simulink model "Project_sim"  (R2025b)
settings: Solver=ode4  StartTime=0.0  StopTime=2*T  FixedStep=0.1  RelTol=1e-3
values from neighbouring files (symbols this model uses):
  a = 3000+R_E    [RUN_ME.m]
  A_0 = [cos(th0+epsilon1) sin(th0+epsilon1) 0; -sin(th0+epsilon1) cos(th0+epsilon1) 0; 0 0 1]*    [1 0 0; 0 cos(i+epsilon2) sin(i+epsilon2); 0 -sin(i+epsilon2) cos(i+epsilon2)]    [RUN_ME.m]
  alpha1 = 0.72    [RUN_ME.m]
  alpha_G0 = 0    [RUN_ME.m]
  AU = astroConstants(2)    [RUN_ME.m]
  b_gyro = deg2rad(0.01*rand(1))    [RUN_ME.m]
  b_mag = 15e-9    (= 1.5e-08)    [RUN_ME.m]
  b_sun = deg2rad(0.1*rand(1))    [RUN_ME.m]
  c_time = 100    [RUN_ME.m]
  D = zeros(3)    [RUN_ME.m]
  den_cz_mag = double(sym2poly(den8_z_mag))    [RUN_ME.m]
  den_cz_sun = double(sym2poly(den8_z_sun))    [RUN_ME.m]
  e = 0.2    [RUN_ME.m]
  epsilon = astroConstants(8)    [RUN_ME.m]
  g_IGRF = [ ... (first row only)    [RUN_ME.m]
  gyro_delay = 1    [RUN_ME.m]
  gyro_mounting = eye(3)    [RUN_ME.m]
  h_IGRF = [ ... (first row only)    [RUN_ME.m]
  I = [Ix 0 0; 0 Iy 0; 0 0 Iz]    [RUN_ME.m]
  i = deg2rad(30)    [RUN_ME.m]
  j_B = [0.01; 0.05; 0.01]    [RUN_ME.m]
  K = place(A, -B, a_controlled)    [RUN_ME.m]
  k1 = 20e-4    (= 0.002)    [RUN_ME.m]
  k1_tilde = 5e-4    (= 0.0005)    [RUN_ME.m]
  k2 = 2e-4    (= 0.0002)    [RUN_ME.m]
  Mis_gyro = deg2rad(0.1*rand(3,1))    [RUN_ME.m]
  Mis_mag = deg2rad(0.1*rand(3,1))    [RUN_ME.m]
  Mis_sun = deg2rad(0.1*rand(3,1))    [RUN_ME.m]
  mu = astroConstants(13)    [RUN_ME.m]
  n = sqrt(mu/a^3)    [RUN_ME.m]
  noise_density_mag = 16e-9    (= 1.6e-08)    [RUN_ME.m]
  Nonorthog_err_gyro = deg2rad(0.1*rand(3,1))    [RUN_ME.m]
  Nonorthog_err_mag = deg2rad(1)*ones(3,1)    [RUN_ME.m]
  num_cz_mag = double(sym2poly(num8_z_mag))    [RUN_ME.m]
  num_cz_sun = double(sym2poly(num8_z_sun))    [RUN_ME.m]
  R_E = astroConstants(23)    [RUN_ME.m]
  R_sun = astroConstants(3)    [RUN_ME.m]
  saturation_gyro = deg2rad(100)    [RUN_ME.m]
  saturation_mag = 60e-6    (= 6e-05)    [RUN_ME.m]
  SF = deg2rad(20*5.25e-3)    [RUN_ME.m]
  SFn = 0.02/100    (= 0.0002)    [RUN_ME.m]
  sigma_ARW = ARW/sqrt(Ts_gyro)    [RUN_ME.m]
  sigma_bias = bias_instability/sqrt(Ts_gyro)    [RUN_ME.m]
  sigma_RRW = RRW/sqrt(Ts_gyro)    [RUN_ME.m]
  sigma_sun = deg2rad(0.5)    [RUN_ME.m]
  th0 = deg2rad(0)    [RUN_ME.m]
  Ts = 0.1    [RUN_ME.m]
  Ts_gyro = 0.1    [RUN_ME.m]
  Ts_mag = 0.1    [RUN_ME.m]
  Ts_sun = 0.1    [RUN_ME.m]
  w_E = 2*pi/T_E    [RUN_ME.m]
  wx_0 = rand(1)*pi/6    [RUN_ME.m]
  wy_0 = rand(1)*pi/6    [RUN_ME.m]
  wz_0 = rand(1)*pi/6    [RUN_ME.m]
undefined symbols (not defined in the file or in its folder): DiscIntNeverNeededParam, dspblkCoreblockFVToolHelper, gcbh, magnitude, precision_sun, RW
libraries: Lib_rotation_matrix x17, matrix_library x11, simulink x3
(part 1 of 3)
settings Model: Creator=stefa  LastModifiedBy=Admin
settings DebuggingCC: MergeDetectMultiDrivingBlocksExec=none
settings ModelReferenceCC: PropagateSignalLabelsOutOfModel=off

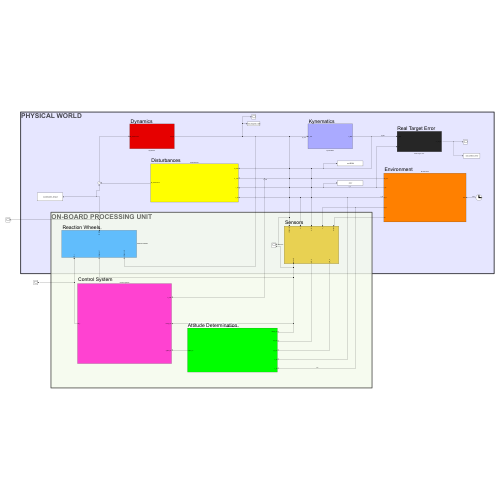
[thumbnail: Simulink's stored preview of the top-level diagram]
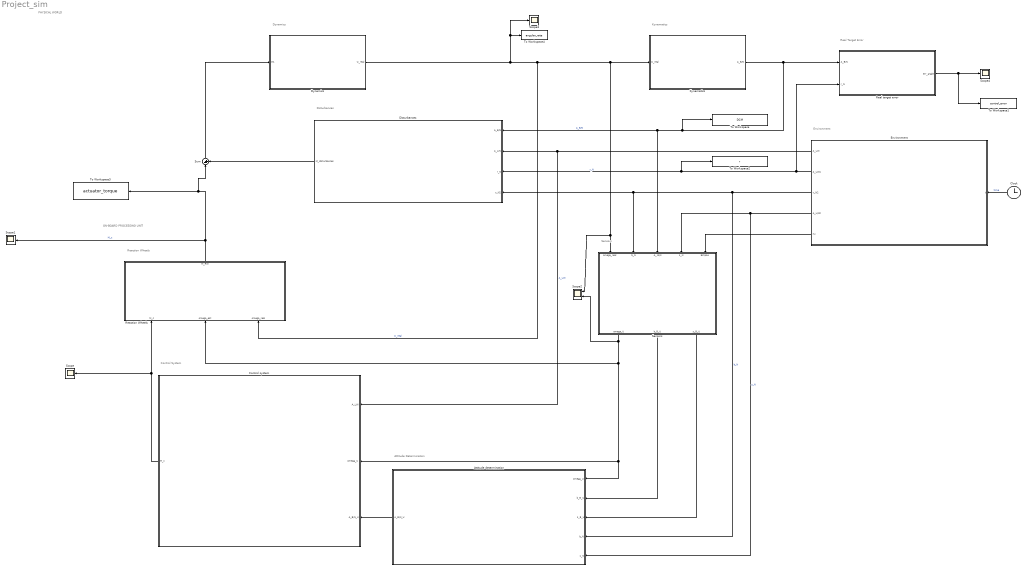
== system Project_sim ==
  note: Attitude Determination
  note: Control System
  note: ON-BOARD PROCESSING UNIT
  note: PHYSICAL WORLD
  note: Sensors
  note: Reaction Wheels
  note: Kynematics
  note: Real Target Error
  note: Environment
  note: Dynamics
  note: Disturbances
  Attitude determination : Subsystem
  Clock : Clock
  Control system : Subsystem
  Disturbances : Subsystem
  Dynamics : Subsystem
  Environment : Subsystem
  Kynematics : Subsystem
  Reaction Wheels : Subsystem
  Real target error : Subsystem
  Scope{,1,3..4} (4 alike) : Scope
      Scope settings: ActiveDisplayYMinimum=-1  ActiveDisplayYMaximum=1  DataLoggingSaveFormat=Array
      Scope1 settings: ActiveDisplayYMinimum=-0.001841  ActiveDisplayYMaximum=0.0018502  DataLoggingSaveFormat=Array
      Scope3 settings: ActiveDisplayYMinimum=-0.075628876788402244  ActiveDisplayYMaximum=0.064125537055305659
      Scope4 settings: ActiveDisplayYMinimum=-0.046604707712651461  ActiveDisplayYMaximum=0.046050366148207011  DataLoggingVariableName=ScopeData4  DataLoggingSaveFormat=Array
  Scope2 : Scope  NumInputPorts=2
      settings: DataLoggingVariableName=ScopeData5  DataLoggingSaveFormat=Array
  Sensors : Subsystem
  Sum : Sum  Inputs=|-+
  To Workspace : ToWorkspace  VariableName=DCM  SampleTime=-1
  To Workspace1 : ToWorkspace  VariableName=control_error  SampleTime=-1
      settings: Save2DSignal=2-D array (concatenate along first dimension)
  To Workspace2 : ToWorkspace  VariableName=r  SampleTime=-1
  To Workspace3 : ToWorkspace  VariableName=actuator_torque  SampleTime=-1
  To Workspace4 : ToWorkspace  VariableName=angular_rate  SampleTime=-1
  wires:
  Dynamics/1(w_real) -> To Workspace4/1, Scope3/1, Kynematics/1(w_real), Scope2/1, Sensors/1(omega_real), Reaction Wheels/3(omega_real)  "w_real"
  Clock/1 -> Environment/1(t)  "time"
  Environment/1(A_L/N) -> Control system/1(A_L/N), Disturbances/2(A_L/N)  "A_L/N"
  Environment/4(A_L/N2) -> Attitude determination/5(s_N), Sensors/4(s_N)  "s_N"
  Environment/3(v_N2) -> Attitude determination/4(b_N), Disturbances/4(v_N2), Sensors/2(b_N)  "b_N"
  Disturbances/1(M_disturbances) -> Sum/2
  Sum/1 -> Dynamics/1(In1)
  Kynematics/1(A_B/N) -> Disturbances/1(A_B/N), Sensors/3(A_ B/N), To Workspace/1, Real target error/1(A_B/N)  "A_B/N"
  Environment/2(A_L/N1) -> Disturbances/3(r_N), To Workspace2/1, Real target error/2(r_N)  "r_N"
  Reaction Wheels/1(M_RW) -> Scope1/1, Sum/1, To Workspace3/1  "M_c"
  Real target error/1(err_angle) -> To Workspace1/1, Scope4/1
  Control system/1(M_c) -> Scope/1, Reaction Wheels/1(M_c)
  Attitude determination/1(A_B/N_U) -> Control system/3(A_B/N_U)
  Sensors/1(omega_U) -> Scope2/2, Reaction Wheels/2(omega_est), Control system/2(omega_U), Attitude determination/1(omega_U)
  Environment/5(nu) -> Sensors/5(Eclipse)
  Sensors/2(b_B_U) -> Attitude determination/2(b_B_U)
  Sensors/3(s_B_U) -> Attitude determination/3(s_B_U)

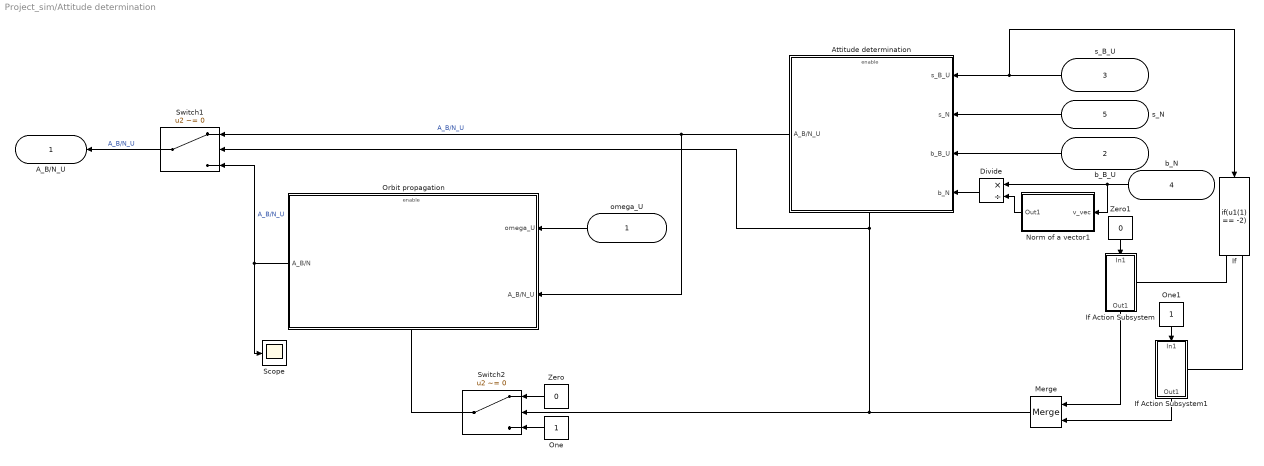
== system Project_sim/Attitude determination ==
  omega_U : Inport
  b_B_U : Inport  Port=2
  s_B_U : Inport  Port=3
  b_N : Inport  Port=4
  s_N : Inport  Port=5
  Attitude determination : Subsystem
  Divide : Product  Inputs=*/
  If : If  IfExpression=u1(1) == -2
  If Action Subsystem : Subsystem  TreatAsAtomicUnit=on
  If Action Subsystem1 : Subsystem  TreatAsAtomicUnit=on
  Merge : Merge
  Norm of a vector1 : Subsystem
  One : Constant  OutDataTypeStr=Inherit: Inherit via back propagation
  One1 : Constant  OutDataTypeStr=Inherit: Inherit via back propagation
  Orbit propagation : Subsystem  TreatAsAtomicUnit=on
  Scope : Scope
      settings: DataLoggingVariableName=ScopeData9  DataLoggingSaveFormat=Array
  Switch1 : Switch  Criteria=u2 ~= 0  SaturateOnIntegerOverflow=off  InputSameDT=off
  Switch2 : Switch  Criteria=u2 ~= 0  SaturateOnIntegerOverflow=off  InputSameDT=off
  Zero : Constant  Value=0  OutDataTypeStr=Inherit: Inherit via back propagation
  Zero1 : Constant  Value=0  OutDataTypeStr=Inherit: Inherit via back propagation
  A_B/N_U : Outport
  wires:
  Switch2/1 -> Orbit propagation/Enable
  b_B_U/1 -> Attitude determination/3(b_B_U)
  omega_U/1 -> Orbit propagation/1(omega_U)
  Attitude determination/1(A_B/N_U) -> Switch1/1, Orbit propagation/2(A_B/N_U)  "A_B/N_U"
  Zero/1 -> Switch2/1
  One/1 -> Switch2/3
  s_B_U/1 -> If/1, Attitude determination/1(s_B_U)
  s_N/1 -> Attitude determination/2(s_N)
  If/1 -> If Action Subsystem/Action
  If/2 -> If Action Subsystem1/Action
  Zero1/1 -> If Action Subsystem/1(In1)
  One1/1 -> If Action Subsystem1/1(In1)
  If Action Subsystem/1(Out1) -> Merge/1
  If Action Subsystem1/1(Out1) -> Merge/2
  Merge/1 -> Switch2/2, Switch1/2, Attitude determination/Enable
  Switch1/1 -> A_B/N_U/1  "A_B/N_U"
  Orbit propagation/1(A_B/N) -> Scope/1, Switch1/3  "A_B/N_U"
  Divide/1 -> Attitude determination/4(b_N)
  b_N/1 -> Norm of a vector1/1(v_vec), Divide/1
  Norm of a vector1/1(Out1) -> Divide/2

== system Project_sim/Control system ==
  A_L/N : Inport
  omega_U : Inport  Port=2
  A_B/N_U : Inport  Port=3
  Control Manager : Subsystem
  Non linear control : Subsystem
  Scope2 : Scope
      settings: ActiveDisplayYMinimum=-0.19795  ActiveDisplayYMaximum=0.17887  DataLoggingVariableName=ScopeData7
  State of system : Subsystem
  Switch2 : Switch  Threshold=1  SaturateOnIntegerOverflow=off  InputSameDT=off
  Switch3 : Switch  Threshold=1  SaturateOnIntegerOverflow=off  InputSameDT=off
  omegaB_nadir : Subsystem
  M_c : Outport
  wires:
  A_L/N/1 -> State of system/3(A_B|N_target), State of system/2(A_L/N), Non linear control/3(A_B/N_target), omegaB_nadir/1(A_L/N)
  omega_U/1 -> State of system/5(omega_U), Control Manager/1(angular velocity), Non linear control/1(omega_U)
  A_B/N_U/1 -> State of system/4(A_B|N_U1), Non linear control/2(A_B/N_U)
  Control Manager/1(First switch) -> Switch2/2
  Control Manager/2(Second switch) -> Switch3/2
  Switch2/1 -> Switch3/3
  Non linear control/2(M_c_detumbling) -> Switch2/3
  Non linear control/3(M_c_repointing) -> Switch2/1
  Switch3/1 -> M_c/1  "M_c"
  Non linear control/1(angle_error) -> Scope2/1, Control Manager/2(angular state)
  omegaB_nadir/1(w_nadir) -> State of system/1(w_nadir), Non linear control/4(w_nadir)
  State of system/1(state) -> Switch3/1

== system Project_sim/Disturbances ==
  A_B/N : Inport
  A_L/N : Inport  Port=2
  r_N : Inport  Port=3
  v_N2 : Inport  Port=4
  Add1 : Sum
  Gravity Gradient : Subsystem
  Magnetic Torque : Subsystem
  M_disturbances : Outport
  wires:
  r_N/1 -> Gravity Gradient/1(A_B/L1)  "r_N"
  A_B/N/1 -> Magnetic Torque/1(A_B|N), Gravity Gradient/2(A_B/L2)  "A_B/N"
  Add1/1 -> M_disturbances/1  "M_disturbances"
  A_L/N/1 -> Gravity Gradient/3(A_B/L3)  "A_L/N"
  Magnetic Torque/1(M_B) -> Add1/1  "M_B"
  Gravity Gradient/1(M_GG) -> Add1/2  "M_GG"
  v_N2/1 -> Magnetic Torque/2(In1)  "b_N"

== system Project_sim/Dynamics ==
  In1 : Inport
  Add1 : Sum
  Constant : Constant  Value=I  VectorParams1D=off
  Cross Product : matrix_library/Cross Product
  Gain : Gain  Gain=inv(I)  Multiplication=Matrix(K*u) (u vector)
  Integrator : Integrator  InitialCondition=[wx_0; wy_0; wz_0]
  Product : Product  Multiplication=Matrix(*)
  w_real : Outport
  wires:
  Add1/1 -> Gain/1
  Gain/1 -> Integrator/1  "omega_dot"
  Integrator/1 -> Cross Product/2, Product/2, w_real/1  "omega"
  Product/1 -> Cross Product/1  "I*omega"
  Cross Product/1 -> Add1/1
  Constant/1 -> Product/1
  In1/1 -> Add1/2  "M_disturbances"

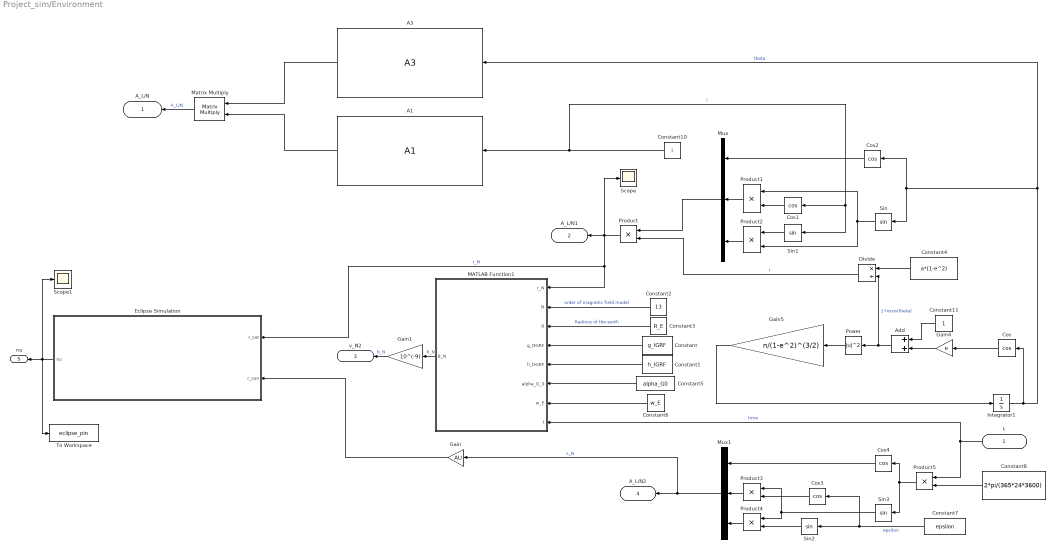
== system Project_sim/Environment ==
  t : Inport
  A1 : Lib_rotation_matrix/A1  SystemSampleTime=-1  VariantActivationTime=update diagram  EmptyChoice=off  PassThrough=off  PassThroughVariantControl=(default)  EmptyChoiceVariantControl=(default)  AllowFlexibleInterface=on  Latency=0  AutoFrameSizeCalculation=off
  A3 : Lib_rotation_matrix/A3  SystemSampleTime=-1  VariantActivationTime=update diagram  EmptyChoice=off  PassThrough=off  PassThroughVariantControl=(default)  EmptyChoiceVariantControl=(default)  AllowFlexibleInterface=on  Latency=0  AutoFrameSizeCalculation=off
  Add : Sum
  Constant : Constant  Value=g_IGRF
  Constant1 : Constant  Value=h_IGRF
  Constant10 : Constant  Value=i
  Constant11 : Constant
  Constant2 : Constant  Value=13
  Constant3 : Constant  Value=R_E
  Constant4 : Constant  Value=a*(1-e^2)
  Constant5 : Constant  Value=alpha_G0
  Constant6 : Constant  Value=w_E
  Constant7 : Constant  Value=epsilon
  Constant8 : Constant  Value=2*pi/(365*24*3600)
  Cos{,1..4} (5 alike) : Trigonometry  Operator=cos
  Divide : Product  Inputs=*/
  Eclipse Simulation : Subsystem
  Gain : Gain  Gain=AU
  Gain1 : Gain  Gain=10^(-9)
  Gain4 : Gain  Gain=e
  Gain5 : Gain  Gain=n/(1-e^2)^(3/2)
  Integrator1 : Integrator  InitialCondition=th0
  MATLAB Function1 : MATLAB Function  TreatAsAtomicUnit=on
  Matrix Multiply : Product  Multiplication=Matrix(*)
  Mux : Mux  Inputs=3
  Mux1 : Mux  Inputs=3
  Power : Math  Operator=magnitude^2
  Product{,1..5} (6 alike) : Product
  Scope : Scope
      settings: DataLoggingVariableName=ScopeData16  DataLoggingSaveFormat=Array
  Scope1 : Scope
      settings: ActiveDisplayYMinimum=-1  ActiveDisplayYMaximum=1  DataLoggingVariableName=ScopeData3
  Sin{,1..3} (4 alike) : Trigonometry
  To Workspace : ToWorkspace  VariableName=eclipse_pin  SampleTime=-1
      settings: Save2DSignal=2-D array (concatenate along first dimension)
  A_L/N : Outport
  A_L/N1 : Outport  Port=2
  v_N2 : Outport  Port=3
  A_L/N2 : Outport  Port=4
  nu : Outport  Port=5
  wires:
  Constant11/1 -> Add/1
  Power/1 -> Gain5/1
  Constant4/1 -> Divide/1
  Gain4/1 -> Add/2
  Cos/1 -> Gain4/1
  Add/1 -> Divide/2, Power/1  "1+ecos(theta)"
  Gain5/1 -> Integrator1/1
  Divide/1 -> Product/2  "r"
  Product2/1 -> Mux/3
  Cos1/1 -> Product1/2
  Product1/1 -> Mux/2
  Cos2/1 -> Mux/1
  Sin/1 -> Product2/2, Product1/1
  Sin1/1 -> Product2/1
  A1/1 -> Matrix Multiply/2
  Integrator1/1 -> A3/1, Cos2/1, Sin/1, Cos/1  "theta"
  Matrix Multiply/1 -> A_L/N/1  "A_L/N"
  A3/1 -> Matrix Multiply/1
  Product/1 -> Scope/1, Eclipse Simulation/1(r_sat), MATLAB Function1/1(r_N), A_L/N1/1  "r_N"
  Mux/1 -> Product/1
  Cos3/1 -> Product3/2
  Sin2/1 -> Product4/2
  Mux1/1 -> Gain/1, A_L/N2/1  "s_N"
  t/1 -> Product5/1, MATLAB Function1/8(t)  "time"
  Product4/1 -> Mux1/3
  Constant7/1 -> Cos3/1, Sin2/1  "epsilon"
  Sin3/1 -> Product4/1, Product3/1
  Constant8/1 -> Product5/2
  Product3/1 -> Mux1/2
  Cos4/1 -> Mux1/1
  Product5/1 -> Sin3/1, Cos4/1
  Constant/1 -> MATLAB Function1/4(g_DGRF)
  Constant1/1 -> MATLAB Function1/5(h_DGRF)
  Constant2/1 -> MATLAB Function1/2(N)  "order of magnetic field model"
  Constant3/1 -> MATLAB Function1/3(R)  "Radious of the earth"
  Constant10/1 -> Sin1/1, Cos1/1, A1/1  "i"
  Constant6/1 -> MATLAB Function1/7(w_E)
  Constant5/1 -> MATLAB Function1/6(alpha_G_0)
  Gain/1 -> Eclipse Simulation/2(r_sun)
  Eclipse Simulation/1(nu) -> To Workspace/1, Scope1/1, nu/1
  Gain1/1 -> v_N2/1  "b_N"
  MATLAB Function1/1(B_N) -> Gain1/1  "b_N"

== system Project_sim/Kynematics ==
  w_real : Inport
  Add : Sum
  Constant1 : Constant  Value=0
  Demux : Demux  Outputs=3
  Gain{1..4} (4 alike) : Gain  Gain=-1
  Gain5 : Gain  Gain=3/2
  Gain6 : Gain  Gain=-1/2
  Integrator1 : Integrator  InitialCondition=A_0
  Product1 : Product  Multiplication=Matrix(*)
  Product2 : Product  Multiplication=Matrix(*)
  Product3 : Product  Multiplication=Matrix(*)
  Reshape : Reshape  OutputDimensionality=Customize  OutputDimensions=[3,3]
  Transpose : Math  Operator=transpose
  Vector Concatenate : Concatenate  NumInputs=9  ConcatenateDimension=2
  A_B/N : Outport
  wires:
  Add/1 -> A_B/N/1, Product1/2  "A_B/N"
  Integrator1/1 -> Product3/1, Transpose/1, Product2/2, Gain5/1
  Gain5/1 -> Add/1
  Reshape/1 -> Gain4/1  "[w]^"
  Product1/1 -> Integrator1/1  "A_dot"
  Transpose/1 -> Product2/1
  Product3/1 -> Gain6/1
  Product2/1 -> Product3/2
  Gain6/1 -> Add/2
  Gain4/1 -> Product1/1
  Constant1/1 -> Vector Concatenate/9, Vector Concatenate/5, Vector Concatenate/1
  w_real/1 -> Demux/1
  Demux/3 -> Vector Concatenate/2, Gain2/1  "w_z"
  Vector Concatenate/1 -> Reshape/1
  Gain3/1 -> Vector Concatenate/8
  Gain2/1 -> Vector Concatenate/4
  Demux/2 -> Gain1/1, Vector Concatenate/7  "w_y"
  Demux/1 -> Vector Concatenate/6, Gain3/1  "w_x"
  Gain1/1 -> Vector Concatenate/3

== system Project_sim/Reaction Wheels ==
  M_c : Inport
  omega_est : Inport  Port=2
  omega_real : Inport  Port=3
  Actuator command : Subsystem
  Constant : Constant  Value=RW.A_inv
  Constant1 : Constant  Value=RW.A
  Constant2 : Constant  Value=RW.I
  Constant6 : Constant  Value=RW.mis
  Demux1 : Demux  Outputs=3
  Divide1 : Product  Inputs=*/
  Integrator1 : Integrator  InitialCondition=RW.omega_act_0
  Min torque : DeadZone  LowerValue=-RW.min_torque  UpperValue=RW.min_torque
  Nonlinear dynamics : Subsystem
  Omit sample until settling time : Subsystem
  Product : Product
  Saturation : Subsystem
  Scope1 : Scope
      settings: DataLoggingVariableName=ScopeData2  DataLoggingSaveFormat=Array
  Subsystem2 : Subsystem
  To Workspace : ToWorkspace  VariableName=RW_omega  SampleTime=-1
  M_RW : Outport
  wires:
  Divide1/1 -> Integrator1/1  "omega_RW_dot"
  Constant1/1 -> Actuator command/4(A)
  Integrator1/1 -> Scope1/1, To Workspace/1, Saturation/1(omega_RW)  "omega_RW"
  Actuator command/1(h_r_dot) -> Nonlinear dynamics/2(h_r_dot)
  Constant/1 -> Actuator command/3(A*)
  Constant2/1 -> Divide1/2
  omega_real/1 -> Nonlinear dynamics/1(omega_real)
  Nonlinear dynamics/1(M) -> Saturation/2(M)
  Saturation/1(M*) -> Min torque/1
  M_c/1 -> Actuator command/2(M_c)
  omega_est/1 -> Actuator command/1(omega_est)
  Product/1 -> M_RW/1
  Omit sample until settling time/1(Out1) -> Product/2  "M_c"
  Min torque/1 -> Divide1/1, Product/1
  Demux1/1 -> Subsystem2/1(In1)
  Demux1/3 -> Subsystem2/3(In3)
  Subsystem2/1(A_real) -> Nonlinear dynamics/3(A_real)  "A_real"
  Constant6/1 -> Demux1/1
  Demux1/2 -> Subsystem2/2(In2)

== system Project_sim/Real target error ==
  A_B/N : Inport
  r_N : Inport  Port=2
  Acos1 : Trigonometry  Operator=acos
  Constant : Constant  Value=[1;0; 0]
  Divide3 : Product  Inputs=*/
  Dot Product : DotProduct  OutDataTypeStr=Inherit: Inherit via internal rule
  MatrixMultiply : Product  Multiplication=Matrix(*)
  Norm of a vector3 : Subsystem
  Transpose : Math  Operator=transpose
  err_angle : Outport
  wires:
  MatrixMultiply/1 -> Dot Product/1  "r_N"
  Divide3/1 -> Dot Product/2  "r_N"
  r_N/1 -> Divide3/1, Norm of a vector3/1(v_vec)
  Dot Product/1 -> Acos1/1
  Norm of a vector3/1(Out1) -> Divide3/2
  Transpose/1 -> MatrixMultiply/1
  Constant/1 -> MatrixMultiply/2
  Acos1/1 -> err_angle/1  "err_angle"
  A_B/N/1 -> Transpose/1

== system Project_sim/Sensors ==
  omega_real : Inport
  b_N : Inport  Port=2
  A_ B/N : Inport  Port=3
  s_N : Inport  Port=4
  Eclipse : Inport  Port=5
  Gyroscope : Subsystem
  Magnetometer : Subsystem
  MatrixMultiply : Product  Multiplication=Matrix(*)
  MatrixMultiply1 : Product  Multiplication=Matrix(*)
  Scope3 : Scope  NumInputPorts=2
      settings: DataLoggingVariableName=ScopeData10  DataLoggingSaveFormat=Array
  Sun sensor : Subsystem
  To Workspace : ToWorkspace  VariableName=s_B_U  SampleTime=-1
  To Workspace1 : ToWorkspace  VariableName=s_B  SampleTime=-1
  omega_U : Outport
  b_B_U : Outport  Port=2
  s_B_U : Outport  Port=3
  wires:
  Eclipse/1 -> Sun sensor/Enable
  Magnetometer/1(s_B_U) -> b_B_U/1
  omega_real/1 -> Gyroscope/1(Angular rates)
  Gyroscope/1(omega_U) -> omega_U/1
  MatrixMultiply/1 -> Magnetometer/1(v_vec)
  b_N/1 -> MatrixMultiply/2
  s_N/1 -> MatrixMultiply1/2
  A_ B/N/1 -> MatrixMultiply1/1, MatrixMultiply/1
  Sun sensor/1(s_B_U) -> s_B_U/1, To Workspace/1, Scope3/2  "s_B_U"
  MatrixMultiply1/1 -> Scope3/1, Sun sensor/1(In1), To Workspace1/1

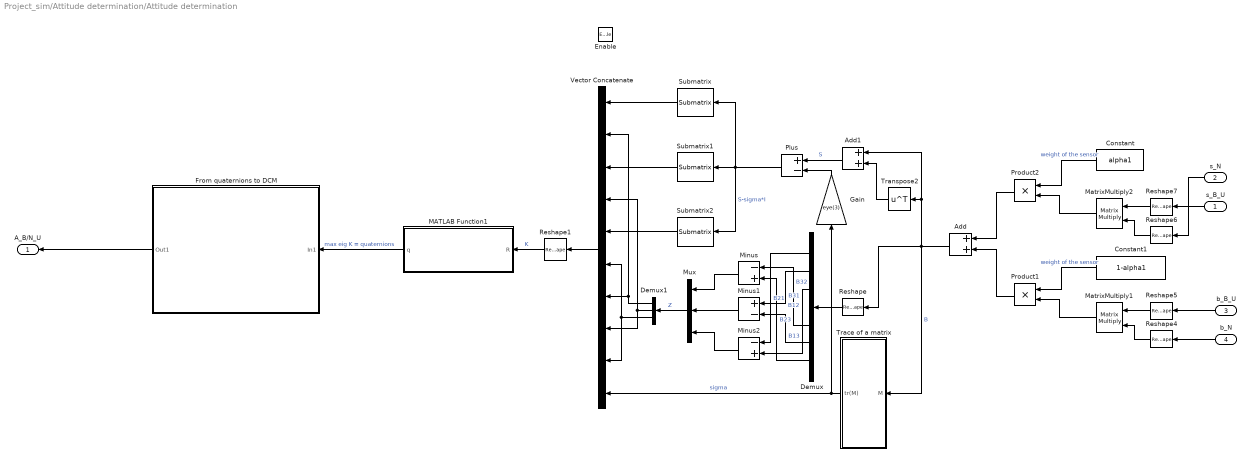
== system Project_sim/Attitude determination/Attitude determination ==
  s_B_U : Inport
  s_N : Inport  Port=2
  b_B_U : Inport  Port=3
  b_N : Inport  Port=4
  Enable : EnablePort  StatesWhenEnabling=reset
  Add : Sum
  Add1 : Sum
  Constant : Constant  Value=alpha1
  Constant1 : Constant  Value=1-alpha1
  Demux : Demux  Outputs=9
  Demux1 : Demux  Outputs=3
  From quaternions to DCM : Subsystem
  Gain : Gain  Gain=eye(3)
  MATLAB Function1 : MATLAB Function  TreatAsAtomicUnit=on
  MatrixMultiply1 : Product  Multiplication=Matrix(*)
  MatrixMultiply2 : Product  Multiplication=Matrix(*)
  Minus : Sum  Inputs=-+
  Minus1 : Sum  Inputs=+-
  Minus2 : Sum  Inputs=-+
  Mux : Mux  Inputs=3
  Plus : Sum  Inputs=+-
  Product1 : Product
  Product2 : Product
  Reshape : Reshape  OutputDimensionality=Column vector (2-D)
  Reshape1 : Reshape  OutputDimensionality=Customize  OutputDimensions=[4,4]
  Reshape4 : Reshape  OutputDimensionality=Row vector (2-D)
  Reshape5 : Reshape  OutputDimensionality=Column vector (2-D)
  Reshape6 : Reshape  OutputDimensionality=Row vector (2-D)
  Reshape7 : Reshape  OutputDimensionality=Column vector (2-D)
  Submatrix : matrix_library/Submatrix  RowSpan=All rows  RowStartMode=First  RowStartIndex=1  RowEndMode=Last  RowEndIndex=1  ColSpan=One column  ColStartMode=First  ColStartIndex=1  ColEndMode=Last  ColEndIndex=1
  Submatrix1 : matrix_library/Submatrix  RowSpan=All rows  RowStartMode=First  RowStartIndex=1  RowEndMode=Last  RowEndIndex=1  ColSpan=One column  ColStartMode=Index  ColStartIndex=2  ColEndMode=Last  ColEndIndex=1
  Submatrix2 : matrix_library/Submatrix  RowSpan=All rows  RowStartMode=First  RowStartIndex=1  RowEndMode=Last  RowEndIndex=1  ColSpan=One column  ColStartMode=Last  ColStartIndex=1  ColEndMode=Last  ColEndIndex=1
  Trace of a matrix : Subsystem
  Transpose2 : Math  Operator=transpose
  Vector Concatenate : Concatenate  NumInputs=10
  A_B/N_U : Outport
  wires:
  Add/1 -> Trace of a matrix/1(M), Transpose2/1, Add1/1, Reshape/1  "B"
  Trace of a matrix/1(tr(M)) -> Vector Concatenate/10, Gain/1  "sigma"
  Transpose2/1 -> Add1/2
  Reshape4/1 -> MatrixMultiply1/2
  b_N/1 -> Reshape4/1
  Reshape/1 -> Demux/1
  Demux/6 -> Minus/1  "B32"
  Demux/8 -> Minus/2  "B23"
  Demux/3 -> Minus1/1  "B31"
  Demux/7 -> Minus1/2  "B13"
  Demux/4 -> Minus2/2  "B12"
  Demux/2 -> Minus2/1  "B21"
  Minus1/1 -> Mux/2
  Minus/1 -> Mux/1
  Minus2/1 -> Mux/3
  Mux/1 -> Demux1/1  "Z"
  Submatrix/1 -> Vector Concatenate/1
  Demux1/1 -> Vector Concatenate/2, Vector Concatenate/7
  Submatrix1/1 -> Vector Concatenate/3
  Demux1/2 -> Vector Concatenate/8, Vector Concatenate/4
  Submatrix2/1 -> Vector Concatenate/5
  Demux1/3 -> Vector Concatenate/9, Vector Concatenate/6
  Vector Concatenate/1 -> Reshape1/1
  Reshape5/1 -> MatrixMultiply1/1
  b_B_U/1 -> Reshape5/1
  Plus/1 -> Submatrix1/1, Submatrix2/1, Submatrix/1  "S-sigma*I"
  Gain/1 -> Plus/2
  Add1/1 -> Plus/1  "S"
  MATLAB Function1/1(q) -> From quaternions to DCM/1(In1)  "max eig K = quaternions"
  Reshape1/1 -> MATLAB Function1/1(R)  "K"
  Constant1/1 -> Product1/1  "weight of the sensor"
  MatrixMultiply1/1 -> Product1/2
  Product1/1 -> Add/2
  MatrixMultiply2/1 -> Product2/2
  Reshape7/1 -> MatrixMultiply2/1
  s_N/1 -> Reshape6/1
  s_B_U/1 -> Reshape7/1
  Reshape6/1 -> MatrixMultiply2/2
  Constant/1 -> Product2/1  "weight of the sensor"
  Product2/1 -> Add/1
  From quaternions to DCM/1(Out1) -> A_B/N_U/1

== system Project_sim/Attitude determination/If Action Subsystem ==
  In1 : Inport
  Action Port : ActionPort  ActionPortLabel=if(u1(1) == -2)
  Out1 : Outport
  wires:
  In1/1 -> Out1/1

== system Project_sim/Attitude determination/If Action Subsystem1 ==
  In1 : Inport
  Action Port : ActionPort  ActionPortLabel=else
  Out1 : Outport
  wires:
  In1/1 -> Out1/1

== system Project_sim/Attitude determination/Norm of a vector1 ==
  v_vec : Inport
  Add : Sum  Inputs=+++
  Demux : Demux  Outputs=3
  Magnitude Squared : Math  Operator=magnitude^2
  Magnitude Squared1 : Math  Operator=magnitude^2
  Magnitude Squared2 : Math  Operator=magnitude^2
  Square Root : Sqrt
  Out1 : Outport
  wires:
  Square Root/1 -> Out1/1  "norm(v)"
  Magnitude Squared2/1 -> Add/3
  Demux/3 -> Magnitude Squared2/1
  Add/1 -> Square Root/1
  Demux/1 -> Magnitude Squared/1
  Magnitude Squared/1 -> Add/1
  Magnitude Squared1/1 -> Add/2
  Demux/2 -> Magnitude Squared1/1
  v_vec/1 -> Demux/1  "v_vec"

== system Project_sim/Attitude determination/Orbit propagation ==
  omega_U : Inport
  A_B/N_U : Inport  Port=2
  Enable : EnablePort  StatesWhenEnabling=reset  ShowOutputPort=on
  Add : Sum
  Constant1 : Constant  Value=0
  Demux : Demux  Outputs=3
  Discrete-Time Integrator : DiscreteIntegrator  ExternalReset=rising  InitialConditionSource=external  SampleTime=-1  ICPrevOutput=DiscIntNeverNeededParam  ICPrevScaledInput=DiscIntNeverNeededParam
  Gain{1..4} (4 alike) : Gain  Gain=-1
  Gain5 : Gain  Gain=3/2
  Gain6 : Gain  Gain=-1/2
  Product1 : Product  Multiplication=Matrix(*)
  Product2 : Product  Multiplication=Matrix(*)
  Product3 : Product  Multiplication=Matrix(*)
  Reshape : Reshape  OutputDimensionality=Customize  OutputDimensions=[3,3]
  Transpose : Math  Operator=transpose
  Vector Concatenate : Concatenate  NumInputs=9  ConcatenateDimension=2
  A_B/N : Outport  OutputWhenDisabled=reset  InitialOutput=0
  wires:
  Product3/1 -> Gain6/1
  Demux/1 -> Vector Concatenate/6, Gain3/1  "w_x"
  A_B/N_U/1 -> Discrete-Time Integrator/3
  Gain6/1 -> Add/2
  Discrete-Time Integrator/1 -> Product3/1, Transpose/1, Product2/2, Gain5/1
  Gain1/1 -> Vector Concatenate/3
  omega_U/1 -> Demux/1
  Product1/1 -> Discrete-Time Integrator/1  "A_dot"
  Add/1 -> A_B/N/1, Product1/2  "A_B/N_U"
  Gain4/1 -> Product1/1
  Transpose/1 -> Product2/1
  Gain2/1 -> Vector Concatenate/4
  Product2/1 -> Product3/2
  Constant1/1 -> Vector Concatenate/9, Vector Concatenate/5, Vector Concatenate/1
  Demux/2 -> Gain1/1, Vector Concatenate/7  "w_y"
  Vector Concatenate/1 -> Reshape/1
  Gain3/1 -> Vector Concatenate/8
  Reshape/1 -> Gain4/1  "[w]^"
  Gain5/1 -> Add/1
  Demux/3 -> Vector Concatenate/2, Gain2/1  "w_z"
  Enable/1 -> Discrete-Time Integrator/2

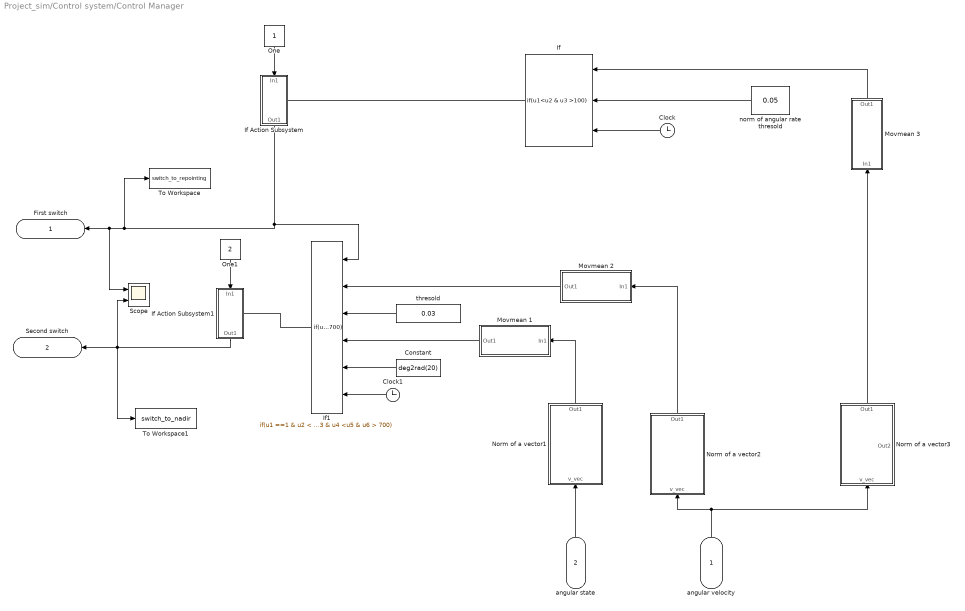
== system Project_sim/Control system/Control Manager ==
  angular velocity : Inport
  angular state : Inport  Port=2
  Clock : Clock
  Clock1 : Clock
      settings: Decimation=1000
  Constant : Constant  Value=deg2rad(20)
  If : If  NumInputs=3  IfExpression=u1<u2 & u3 >100  ShowElse=off
  If Action Subsystem : Subsystem  TreatAsAtomicUnit=on
  If Action Subsystem1 : Subsystem  TreatAsAtomicUnit=on
  If1 : If  NumInputs=6  IfExpression=u1 ==1 & u2 < u3 & u4 <u5 & u6 > 700  ShowElse=off
  Movmean 1 : Subsystem
  Movmean 2 : Subsystem
  Movmean 3 : Subsystem
  Norm of a vector1 : Subsystem
  Norm of a vector2 : Subsystem
  Norm of a vector3 : Subsystem
      settings: PortSchema="{\"entries\":[{\"content\":{\"sides\":[{\"content\":{\"connectorIds\":[\"In1\"]},\"type\":\"ConnectorPlacement.EquallySpacedRectSide\",\"uuid\":\"8ebd8283-d03e-4465-ac96-7f047cb36717\"},{\"content\":{\"connectorIds\":[\"Out1\"],\"side\":\"RIGHT\"},\"type\":\"ConnectorPlacement.EquallySpacedRectSide\",\"uuid\":\"f3f952ac-6300-468b-a1c2-270feabae7f9\"},{\"content\":{\"side\":\"TOP\"},\"type\":\"ConnectorPlacement.EquallySpacedRectSide\",\"uuid\":\"08a2905a-2cb7-49c2-9c88-fdda1c06d68a\"},{\"content\":{\"connectorIds\":[\"Out2\"],\"side\":\"BOTTOM\"},\"type\":\"ConnectorPlacement.EquallySpacedRectSide\",\"uuid\":\"2a15cd15-3cba-48c1-b9fe-4497c7463d1d\"}]},\"type\":\"ConnectorPlacement.EquallySpacedConnector\",\"uuid\":\"2dbf0da0-6f21-44d0-9037-a35afe66e556\"}],\"packageUris\":[\"http://schema.mathworks.com/mf0/Connector/R2020b\"],\"version\":\"1.0\"}"
  One : Constant  OutDataTypeStr=Inherit: Inherit via back propagation
  One1 : Constant  Value=2  OutDataTypeStr=Inherit: Inherit via back propagation
  Scope : Scope  NumInputPorts=2
      settings: ActiveDisplayYMinimum=-0.25  ActiveDisplayYMaximum=2.25  DataLoggingVariableName=ScopeData2  DataLoggingSaveFormat=Array
  To Workspace : ToWorkspace  VariableName=switch_to_repointing  SampleTime=-1
      settings: Save2DSignal=2-D array (concatenate along first dimension)
  To Workspace1 : ToWorkspace  VariableName=switch_to_nadir  SampleTime=-1
      settings: Save2DSignal=2-D array (concatenate along first dimension)
  norm of angular rate thresold : Constant  Value=0.05
  thresold : Constant  Value=0.03
  First switch : Outport
  Second switch : Outport  Port=2
  wires:
  Movmean 3/1(Out1) -> If/1
  One/1 -> If Action Subsystem/1(In1)
  Norm of a vector3/1(Out1) -> Movmean 3/1(In1)
  norm of angular rate thresold/1 -> If/2
  If Action Subsystem/1(Out1) -> To Workspace/1, Scope/1, First switch/1, If1/1
  angular velocity/1 -> Norm of a vector2/1(v_vec), Norm of a vector3/1(v_vec)
  Clock/1 -> If/3
  angular state/1 -> Norm of a vector1/1(v_vec)
  Clock1/1 -> If1/6
  thresold/1 -> If1/3
  Norm of a vector1/1(Out1) -> Movmean 1/1(In1)
  One1/1 -> If Action Subsystem1/1(In1)
  If1/1 -> If Action Subsystem1/Action
  If Action Subsystem1/1(Out1) -> To Workspace1/1, Scope/2, Second switch/1
  Norm of a vector2/1(Out1) -> Movmean 2/1(In1)
  If/1 -> If Action Subsystem/Action
  Movmean 2/1(Out1) -> If1/2
  Movmean 1/1(Out1) -> If1/4
  Constant/1 -> If1/5

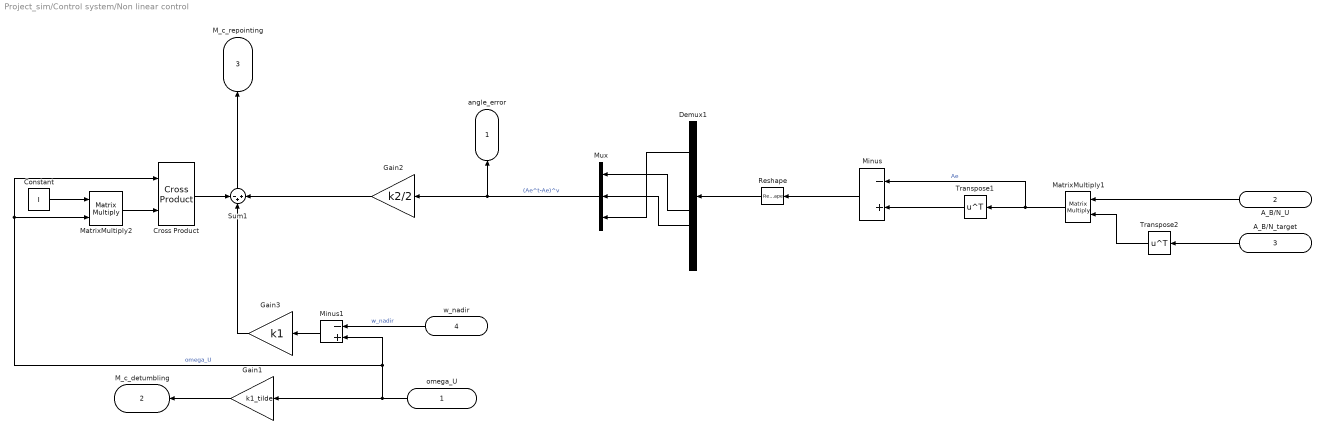
== system Project_sim/Control system/Non linear control ==
  omega_U : Inport
  A_B/N_U : Inport  Port=2
  A_B/N_target : Inport  Port=3
  w_nadir : Inport  Port=4
  Constant : Constant  Value=I
  Cross Product : matrix_library/Cross Product
  Demux1 : Demux  Outputs=9
  Gain1 : Gain  Gain=k1_tilde
  Gain2 : Gain  Gain=k2/2
  Gain3 : Gain  Gain=k1
  MatrixMultiply1 : Product  Multiplication=Matrix(*)
  MatrixMultiply2 : Product  Multiplication=Matrix(*)
  Minus : Sum  Inputs=-+
  Minus1 : Sum  Inputs=-+
  Mux : Mux  Inputs=3
  Reshape : Reshape  OutputDimensionality=Column vector (2-D)
  Sum1 : Sum  Inputs=-++
  Transpose1 : Math  Operator=transpose
  Transpose2 : Math  Operator=transpose
  angle_error : Outport
  M_c_detumbling : Outport  Port=2
  M_c_repointing : Outport  Port=3
  wires:
  Minus/1 -> Reshape/1
  Reshape/1 -> Demux1/1
  Mux/1 -> Gain2/1, angle_error/1  "(Ae^t-Ae)^v"
  Demux1/2 -> Mux/3
  Demux1/7 -> Mux/2
  Gain2/1 -> Sum1/3
  Demux1/6 -> Mux/1
  Transpose1/1 -> Minus/2
  Sum1/1 -> M_c_repointing/1
  A_B/N_target/1 -> Transpose2/1
  Transpose2/1 -> MatrixMultiply1/2
  w_nadir/1 -> Minus1/1  "w_nadir"
  A_B/N_U/1 -> MatrixMultiply1/1
  MatrixMultiply1/1 -> Minus/1, Transpose1/1  "Ae"
  Gain1/1 -> M_c_detumbling/1
  Gain3/1 -> Sum1/2
  Minus1/1 -> Gain3/1
  omega_U/1 -> Cross Product/1, MatrixMultiply2/2, Minus1/2, Gain1/1  "omega_U"
  MatrixMultiply2/1 -> Cross Product/2
  Constant/1 -> MatrixMultiply2/1
  Cross Product/1 -> Sum1/1

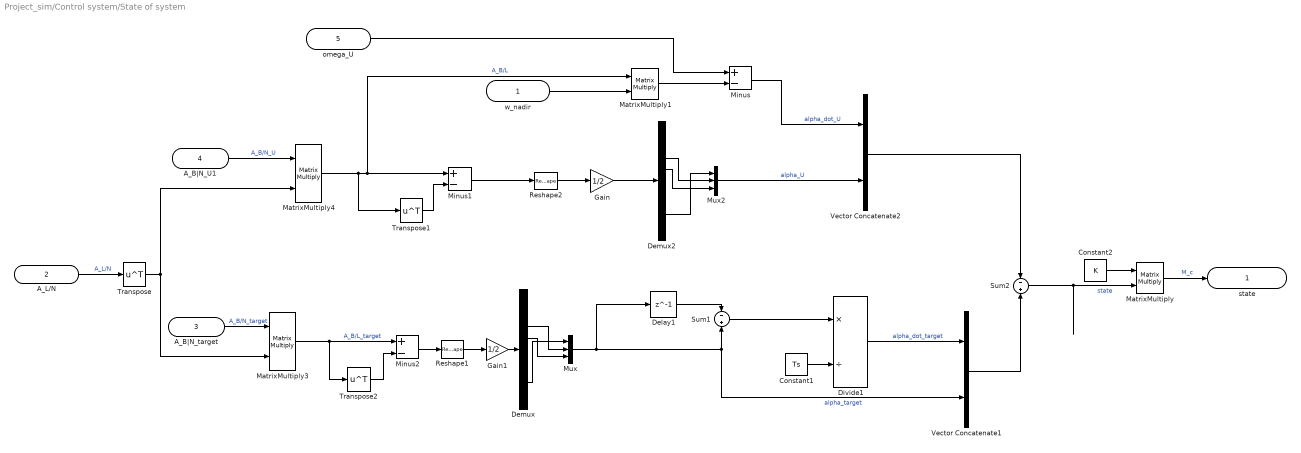
== system Project_sim/Control system/State of system ==
  w_nadir : Inport
  A_L/N : Inport  Port=2
  A_B|N_target : Inport  Port=3
  A_B|N_U1 : Inport  Port=4
  omega_U : Inport  Port=5
  Constant1 : Constant  Value=Ts
  Constant2 : Constant  Value=K
  Delay1 : Delay  DelayLength=1
  Demux : Demux  Outputs=9
  Demux2 : Demux  Outputs=9
  Divide1 : Product  Inputs=*/
  Gain : Gain  Gain=1/2
  Gain1 : Gain  Gain=1/2
  MatrixMultiply{,1,3..4} (4 alike) : Product  Multiplication=Matrix(*)
  Minus : Sum  Inputs=+-
  Minus1 : Sum  Inputs=+-
  Minus2 : Sum  Inputs=+-
  Mux : Mux  Inputs=3
  Mux2 : Mux  Inputs=3
  Reshape1 : Reshape  OutputDimensionality=Column vector (2-D)
  Reshape2 : Reshape  OutputDimensionality=Column vector (2-D)
  Sum1 : Sum  Inputs=-+
  Sum2 : Sum  Inputs=-+
  Transpose : Math  Operator=transpose
  Transpose1 : Math  Operator=transpose
  Transpose2 : Math  Operator=transpose
  Vector Concatenate1 : Concatenate
  Vector Concatenate2 : Concatenate
  state : Outport
  wires:
  A_L/N/1 -> Transpose/1  "A_L/N"
  Vector Concatenate1/1 -> Sum2/2
  Constant1/1 -> Divide1/2
  Sum1/1 -> Divide1/1
  Demux/4 -> Mux/3
  Demux/8 -> Mux/1
  A_B|N_target/1 -> MatrixMultiply3/1  "A_B/N_target"
  Mux/1 -> Vector Concatenate1/2, Sum1/2, Delay1/1  "alpha_target"
  Delay1/1 -> Sum1/1
  Divide1/1 -> Vector Concatenate1/1  "alpha_dot_target"
  Sum2/1 -> MatrixMultiply/2  "state"
  Demux/3 -> Mux/2
  Constant2/1 -> MatrixMultiply/1
  MatrixMultiply/1 -> state/1  "M_c"
  Demux2/4 -> Mux2/3
  Vector Concatenate2/1 -> Sum2/1
  A_B|N_U1/1 -> MatrixMultiply4/1  "A_B/N_U"
  Demux2/8 -> Mux2/1
  Minus/1 -> Vector Concatenate2/1  "alpha_dot_U"
  MatrixMultiply4/1 -> Transpose1/1, Minus1/1, MatrixMultiply1/1  "A_B/L"
  Demux2/3 -> Mux2/2
  Transpose/1 -> MatrixMultiply4/2, MatrixMultiply3/2
  Mux2/1 -> Vector Concatenate2/2  "alpha_U"
  MatrixMultiply1/1 -> Minus/2
  omega_U/1 -> Minus/1
  w_nadir/1 -> MatrixMultiply1/2
  Minus1/1 -> Reshape2/1
  Transpose1/1 -> Minus1/2
  Gain/1 -> Demux2/1
  Gain1/1 -> Demux/1
  Transpose2/1 -> Minus2/2
  MatrixMultiply3/1 -> Minus2/1, Transpose2/1  "A_B/L_target"
  Reshape1/1 -> Gain1/1
  Minus2/1 -> Reshape1/1
  Reshape2/1 -> Gain/1

== system Project_sim/Control system/omegaB_nadir ==
  A_L/N : Inport
  Constant3 : Constant  Value=Ts
  Delay2 : Delay  DelayLength=1
  Demux2 : Demux  Outputs=9
  Divide2 : Product  Inputs=*/
  Gain : Gain  Gain=-1
  MatrixMultiply : Product  Multiplication=Matrix(*)
  Mux1 : Mux  Inputs=3
  Reshape1 : Reshape  OutputDimensionality=Column vector (2-D)
  Reshape2 : Reshape  OutputDimensionality=Customize  OutputDimensions=[3,3]
  Reshape3 : Reshape  OutputDimensionality=Column vector (2-D)
  Sum4 : Sum  Inputs=+-
  Transpose2 : Math  Operator=transpose
  w_nadir : Outport
  wires:
  Delay2/1 -> Sum4/2
  Constant3/1 -> Divide2/2
  Demux2/6 -> Mux1/1
  Transpose2/1 -> MatrixMultiply/2
  Mux1/1 -> Gain/1  "omega_U"
  Reshape3/1 -> Demux2/1
  Demux2/7 -> Mux1/2
  Reshape1/1 -> Sum4/1, Delay2/1
  Demux2/2 -> Mux1/3
  Reshape2/1 -> MatrixMultiply/1  "dA/dt"
  Divide2/1 -> Reshape2/1  "alpha_dot_target"
  MatrixMultiply/1 -> Reshape3/1
  A_L/N/1 -> Transpose2/1, Reshape1/1
  Sum4/1 -> Divide2/1
  Gain/1 -> w_nadir/1  "w_nadir"

== system Project_sim/Disturbances/Gravity Gradient ==
  A_B/L1 : Inport
  A_B/L2 : Inport  Port=2
  A_B/L3 : Inport  Port=3
  Constant : Constant  Value=-3
  Constant2 : Constant
  Constant3 : Constant  Value=0
  Constant9 : Constant  Value=I
  Cross Product1 : matrix_library/Cross Product
  Gain7 : Gain  Gain=3*mu
  Matrix Multiply1 : Product  Multiplication=Matrix(*)
  Matrix Multiply2 : Product  Multiplication=Matrix(*)
  Norm of a vector : Subsystem
  Product : Product
  Product1 : Product  Multiplication=Matrix(*)
  Square : Math  Operator=pow
  Transpose1 : Math  Operator=transpose
  Vector Concatenate1 : Concatenate  NumInputs=3  ConcatenateDimension=2
  M_GG : Outport
  wires:
  Constant9/1 -> Matrix Multiply2/1
  Vector Concatenate1/1 -> Matrix Multiply1/2
  Matrix Multiply1/1 -> Cross Product1/1, Matrix Multiply2/2  "[c1; c2; c3]"
  Constant3/1 -> Vector Concatenate1/3, Vector Concatenate1/2
  Cross Product1/1 -> Gain7/1
  Constant2/1 -> Vector Concatenate1/1
  Matrix Multiply2/1 -> Cross Product1/2  "Ic"
  Product/1 -> M_GG/1  "M_GG"
  Gain7/1 -> Product/2  "M_GG"
  Constant/1 -> Square/2
  Norm of a vector/1(Out1) -> Square/1  "r"
  Square/1 -> Product/1
  A_B/L1/1 -> Norm of a vector/1(v_vec)  "r_N"
  A_B/L3/1 -> Transpose1/1  "A_L/N"
  Transpose1/1 -> Product1/2
  A_B/L2/1 -> Product1/1  "A_B/N"
  Product1/1 -> Matrix Multiply1/1  "A_B/L"

== system Project_sim/Disturbances/Magnetic Torque ==
  A_B|N : Inport
  In1 : Inport  Port=2
  Constant : Constant  Value=j_B
  Cross Product2 : matrix_library/Cross Product
  MatrixMultiply2 : Product  Multiplication=Matrix(*)
  M_B : Outport
  wires:
  Cross Product2/1 -> M_B/1  "M_B"
  In1/1 -> MatrixMultiply2/2  "b_N"
  A_B|N/1 -> MatrixMultiply2/1
  MatrixMultiply2/1 -> Cross Product2/2  "b_B"
  Constant/1 -> Cross Product2/1

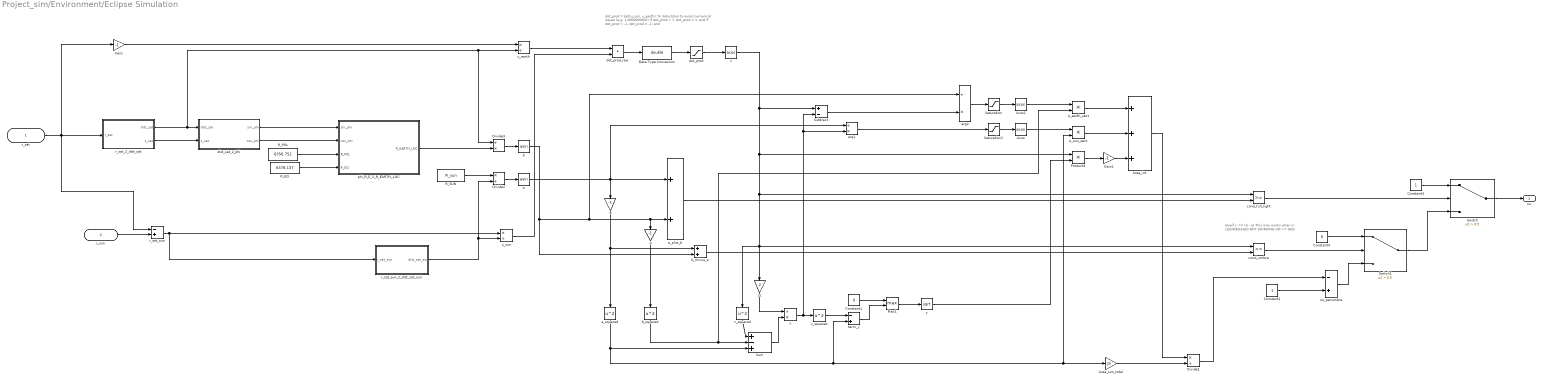
== system Project_sim/Environment/Eclipse Simulation ==
  note: dot_prod = dot(u_sun, u_earth);
      |
      | % Saturation to avoid numerical issues (e.g. 1.0000000002)
      | if dot_prod > 1, dot_prod = 1; end
      | if dot_prod < -1, dot_prod = -1; end
  note: elseif c <= (b - a)
      | This only works when in LEO/MEO/HEO
      | NOT WORKING ON >= GEO
  r_sat : Inport
  r_sun : Inport  Port=2
  -a : Gain  Gain=-1
  -b : Gain  Gain=-1
  2c : Gain  Gain=2
  A_earth_sect : Product
  A_sun_sect : Product
  Acos : Trigonometry  Operator=acos
  Acos1 : Trigonometry  Operator=acos
  Area_int : Sum  Inputs=+++
  Area_sun_total : Gain  Gain=pi
  Constant1 : Constant  Value=0
  Constant2 : Constant
  Constant3 : Constant
  Constant4 : Constant  Value=0
  Data Type Conversion : DataTypeConversion  OutDataTypeStr=double  SaturateOnIntegerOverflow=off  RndMeth=Floor
  Divide1 : Product  Inputs=*/
  Divide2 : Product  Inputs=*/
  Divide3 : Product  Inputs=/*
  Gain : Gain  Gain=-1
  Gain1 : Gain  Gain=-1
  Max1 : MinMax  Function=max  Inputs=2
  Product4 : Product
  R_EQ : Constant  Value=6378.137
  R_POL : Constant  Value=6356.752
  R_SUN : Constant  Value=R_sun
  Saturation : Saturate  UpperLimit=1  LowerLimit=-1
  Saturation1 : Saturate  UpperLimit=1  LowerLimit=-1
  Subtract : Sum  Inputs=+-
  Sum : Sum  Inputs=+-+
  Switch : Switch  Criteria=u2 > Threshold  Threshold=0.5  SaturateOnIntegerOverflow=off  InputSameDT=off
  Switch1 : Switch  Criteria=u2 > Threshold  Threshold=0.5  SaturateOnIntegerOverflow=off  InputSameDT=off
  a : Trigonometry  Operator=asin
  a_plus_b : Sum
  a_squared : Math  Operator=square
  arg1 : Product  Inputs=/*
  arg2 : Product  Inputs=/*
  b : Trigonometry  Operator=asin
  b_minus_a : Sum
  b_squared : Math  Operator=square
  c : Trigonometry  Operator=acos
  c_squared : Math  Operator=square
  cond_full_light : RelationalOperator  OutDataTypeStr=boolean  RndMeth=Simplest  InputSameDT=off
  cond_umbra : RelationalOperator  Operator=<=  OutDataTypeStr=boolean  RndMeth=Simplest  InputSameDT=off
  dist_sat_2_phi : Subsystem
  dot_prod : Saturate  UpperLimit=1  LowerLimit=-1
  dot_prod_raw : DotProduct  OutDataTypeStr=Inherit: Inherit via internal rule
  nu_penumbra : Sum  Inputs=-+
  phi_R_E_2_R_EARTH_LOC : Subsystem
  r_sat_2_dist_sat : Subsystem
  r_sat_sun : Sum  Inputs=-+
  r_sat_sun_2_dist_sat_sun : Subsystem
  term_y : Sum  Inputs=-+
  u_earth : Product  Inputs=*/
  u_sun : Product  Inputs=*/
  x : Product  Inputs=/*
  x_squared : Math  Operator=square
  y : Sqrt
  nu : Outport
  wires:
  Acos1/1 -> A_earth_sect/1
  Constant2/1 -> nu_penumbra/2
  Area_int/1 -> Divide1/1
  Constant3/1 -> Switch/1
  r_sat_sun/1 -> r_sat_sun_2_dist_sat_sun/1(r_sat_sun), u_sun/1
  -b/1 -> b_squared/1
  r_sun/1 -> r_sat_sun/2
  x_squared/1 -> term_y/1
  Constant4/1 -> Switch1/1
  Sum/1 -> x/2
  -a/1 -> a_squared/1, b_minus_a/1
  Subtract/1 -> arg2/2
  Saturation/1 -> Acos1/1
  cond_umbra/1 -> Switch1/2
  b/1 -> b_minus_a/2, -b/1, a_plus_b/2, arg2/1
  c_squared/1 -> Sum/1
  Gain/1 -> u_earth/1
  a_plus_b/1 -> cond_full_light/2
  y/1 -> Product4/2
  Product4/1 -> Gain1/1
  arg2/1 -> Saturation/1
  Gain1/1 -> Area_int/3
  dot_prod/1 -> c/1
  2c/1 -> x/1
  Saturation1/1 -> Acos/1
  Divide1/1 -> nu_penumbra/1
  r_sat/1 -> Gain/1, r_sat_sun/1, r_sat_2_dist_sat/1(r_sat)
  a_squared/1 -> A_sun_sect/2, Area_sun_total/1, term_y/2, Sum/3
  b_minus_a/1 -> cond_umbra/2
  u_earth/1 -> dot_prod_raw/1
  Area_sun_total/1 -> Divide1/2
  R_SUN/1 -> Divide2/1
  c/1 -> Product4/1, 2c/1, c_squared/1, cond_umbra/1, cond_full_light/1, Subtract/1
  Switch/1 -> nu/1
  Max1/1 -> y/1
  Divide2/1 -> a/1
  Divide3/1 -> b/1
  A_sun_sect/1 -> Area_int/2
  cond_full_light/1 -> Switch/2
  Data Type Conversion/1 -> dot_prod/1
  u_sun/1 -> dot_prod_raw/2
  Acos/1 -> A_sun_sect/1
  term_y/1 -> Max1/2
  arg1/1 -> Saturation1/1
  Constant1/1 -> Max1/1
  x/1 -> x_squared/1, arg1/2, Subtract/2
  Switch1/1 -> Switch/3
  b_squared/1 -> Sum/2, A_earth_sect/2
  nu_penumbra/1 -> Switch1/3
  dot_prod_raw/1 -> Data Type Conversion/1
  a/1 -> -a/1, arg1/1, a_plus_b/1
  A_earth_sect/1 -> Area_int/1
  r_sat_2_dist_sat/1(dist_sat) -> u_earth/2, Divide3/1, dist_sat_2_phi/1(dist_sat)
  r_sat_2_dist_sat/2(z_sat) -> dist_sat_2_phi/2(z_sat)
  dist_sat_2_phi/1(sin_phi) -> phi_R_E_2_R_EARTH_LOC/1(sin_phi)
  dist_sat_2_phi/2(cos_phi) -> phi_R_E_2_R_EARTH_LOC/2(cos_phi)
  R_POL/1 -> phi_R_E_2_R_EARTH_LOC/3(R_POL)
  R_EQ/1 -> phi_R_E_2_R_EARTH_LOC/4(R_EQ)
  phi_R_E_2_R_EARTH_LOC/1(R_EARTH_LOC) -> Divide3/2
  r_sat_sun_2_dist_sat_sun/1(dist_sat_sun) -> Divide2/2, u_sun/2

== system Project_sim/Reaction Wheels/Actuator command ==
  omega_est : Inport
  M_c : Inport  Port=2
  A* : Inport  Port=3
  A : Inport  Port=4
  Constant : Constant  Value=I
  Cross Product : matrix_library/Cross Product
  Cross Product1 : matrix_library/Cross Product
  Integrator1 : Integrator
  MatrixMultiply : Product  Multiplication=Matrix(*)
  MatrixMultiply1 : Product  Multiplication=Matrix(*)
  MatrixMultiply2 : Product  Multiplication=Matrix(*)
  Reshape : Reshape  OutputDimensionality=Column vector (2-D)
  Reshape1 : Reshape  OutputDimensionality=Column vector (2-D)
  Sum2 : Sum  Inputs=---
  h_r_dot : Outport
  wires:
  MatrixMultiply1/1 -> Cross Product1/2
  Sum2/1 -> MatrixMultiply2/2
  Integrator1/1 -> MatrixMultiply1/2  "h_r"
  MatrixMultiply/1 -> Cross Product/2
  Constant/1 -> MatrixMultiply/1
  omega_est/1 -> Reshape/1
  MatrixMultiply2/1 -> h_r_dot/1, Integrator1/1  "h_r_dot"
  A*/1 -> MatrixMultiply2/1
  A/1 -> MatrixMultiply1/1
  M_c/1 -> Reshape1/1
  Reshape/1 -> Cross Product/1, Cross Product1/1, MatrixMultiply/2
  Reshape1/1 -> Sum2/1
  Cross Product/1 -> Sum2/2
  Cross Product1/1 -> Sum2/3

== system Project_sim/Reaction Wheels/Nonlinear dynamics ==
  omega_real : Inport
  h_r_dot : Inport  Port=2
  A_real : Inport  Port=3
  Constant : Constant  Value=I
  Cross Product : matrix_library/Cross Product
  Cross Product1 : matrix_library/Cross Product
  Integrator : Integrator
  MatrixMultiply1 : Product  Multiplication=Matrix(*)
  MatrixMultiply2 : Product  Multiplication=Matrix(*)
  MatrixMultiply3 : Product  Multiplication=Matrix(*)
  Sum : Sum  Inputs=---
  M : Outport
  wires:
  Constant/1 -> MatrixMultiply1/1
  omega_real/1 -> Cross Product1/1, MatrixMultiply1/2, Cross Product/1
  MatrixMultiply1/1 -> Cross Product/2
  A_real/1 -> MatrixMultiply2/1, MatrixMultiply3/1
  h_r_dot/1 -> Integrator/1, MatrixMultiply2/2
  Integrator/1 -> MatrixMultiply3/2
  MatrixMultiply3/1 -> Cross Product1/2
  Sum/1 -> M/1
  MatrixMultiply2/1 -> Sum/2
  Cross Product1/1 -> Sum/3
  Cross Product/1 -> Sum/1

== system Project_sim/Reaction Wheels/Omit sample until settling time ==
  Clock : Clock
  If : If  IfExpression=u1 <= Ts
  If Action Subsystem : Subsystem  TreatAsAtomicUnit=on
  If Action Subsystem1 : Subsystem  TreatAsAtomicUnit=on
  Merge : Merge
  Out1 : Outport
  wires:
  If Action Subsystem1/1(Out1) -> Merge/2
  If Action Subsystem/1(Out1) -> Merge/1
  If/2 -> If Action Subsystem1/Action
  Merge/1 -> Out1/1
  If/1 -> If Action Subsystem/Action
  Clock/1 -> If/1

== system Project_sim/Reaction Wheels/Saturation ==
  omega_RW : Inport
  M : Inport  Port=2
  Demux : Demux  Outputs=3
  Demux1 : Demux  Outputs=3
  Gain : Gain  Gain=-1
  Gain1 : Gain  Gain=-1
  Gain2 : Gain  Gain=-1
  Max_torque(omega) : Subsystem  AncestorBlock=SAD/Reaction wheel/Max_torque(omega)
  Max_torque(omega)1 : Subsystem  AncestorBlock=SAD/Reaction wheel/Max_torque(omega)
  Max_torque(omega)2 : Subsystem  AncestorBlock=SAD/Reaction wheel/Max_torque(omega)
  Mux : Mux  Inputs=3
  RW saturation : simulink/Discontinuities/Saturation Dynamic  OutMin=[]  OutMax=[]  OutDataTypeStr=Inherit: Same as second input  OutDataType=fixdt(1, 16)  OutScaling=2^-10  DoSatur=off
  RW saturation1 : simulink/Discontinuities/Saturation Dynamic  OutMin=[]  OutMax=[]  OutDataTypeStr=Inherit: Same as second input  OutDataType=fixdt(1, 16)  OutScaling=2^-10  DoSatur=off
  RW saturation2 : simulink/Discontinuities/Saturation Dynamic  OutMin=[]  OutMax=[]  OutDataTypeStr=Inherit: Same as second input  OutDataType=fixdt(1, 16)  OutScaling=2^-10  DoSatur=off
  Reshape : Reshape  OutputDimensionality=Column vector (2-D)
  Reshape1 : Reshape  OutputDimensionality=Column vector (2-D)
  Reshape2 : Reshape  OutputDimensionality=Column vector (2-D)
  M* : Outport
  wires:
  M/1 -> Reshape1/1
  Reshape/1 -> M*/1
  Demux/1 -> RW saturation1/2
  Demux/2 -> RW saturation2/2
  Demux/3 -> RW saturation/2
  RW saturation1/1 -> Mux/1
  RW saturation2/1 -> Mux/2
  RW saturation/1 -> Mux/3
  Mux/1 -> Reshape/1
  Gain2/1 -> RW saturation/3
  Gain1/1 -> RW saturation2/3
  Gain/1 -> RW saturation1/3
  Max_torque(omega)/1(M_max) -> Gain/1, RW saturation1/1
  Max_torque(omega)1/1(M_max) -> RW saturation2/1, Gain1/1
  Max_torque(omega)2/1(M_max) -> RW saturation/1, Gain2/1
  Demux1/3 -> Max_torque(omega)2/1(omega_RW)
  Demux1/2 -> Max_torque(omega)1/1(omega_RW)
  Demux1/1 -> Max_torque(omega)/1(omega_RW)
  omega_RW/1 -> Reshape2/1
  Reshape1/1 -> Demux/1
  Reshape2/1 -> Demux1/1

== system Project_sim/Reaction Wheels/Subsystem2 ==
  In1 : Inport
  In2 : Inport  Port=2
  In3 : Inport  Port=3
  A1 : Lib_rotation_matrix/A1  SystemSampleTime=-1  VariantActivationTime=update diagram  EmptyChoice=off  PassThrough=off  PassThroughVariantControl=(default)  EmptyChoiceVariantControl=(default)  AllowFlexibleInterface=on  Latency=0  AutoFrameSizeCalculation=off
  A2 : Lib_rotation_matrix/A2  SystemSampleTime=-1  VariantActivationTime=update diagram  EmptyChoice=off  PassThrough=off  PassThroughVariantControl=(default)  EmptyChoiceVariantControl=(default)  AllowFlexibleInterface=on  Latency=0  AutoFrameSizeCalculation=off
  A3 : Lib_rotation_matrix/A3  SystemSampleTime=-1  VariantActivationTime=update diagram  EmptyChoice=off  PassThrough=off  PassThroughVariantControl=(default)  EmptyChoiceVariantControl=(default)  AllowFlexibleInterface=on  Latency=0  AutoFrameSizeCalculation=off
  MatrixMultiply : Product  Multiplication=Matrix(*)
  MatrixMultiply1 : Product  Multiplication=Matrix(*)
  A_real : Outport
  wires:
  MatrixMultiply/1 -> MatrixMultiply1/1
  A3/1 -> MatrixMultiply1/2
  A1/1 -> MatrixMultiply/1
  MatrixMultiply1/1 -> A_real/1  "A_real"
  A2/1 -> MatrixMultiply/2
  In1/1 -> A1/1  "amplitude of misalignment x"
  In2/1 -> A2/1  "amplitude of misalignment y"
  In3/1 -> A3/1  "amplitude of misalignment z"

== system Project_sim/Real target error/Norm of a vector3 ==
  v_vec : Inport
  Add : Sum  Inputs=+++
  Demux : Demux  Outputs=3
  Magnitude Squared : Math  Operator=magnitude^2
  Magnitude Squared1 : Math  Operator=magnitude^2
  Magnitude Squared2 : Math  Operator=magnitude^2
  Square Root : Sqrt
  Out1 : Outport
  wires:
  Square Root/1 -> Out1/1  "norm(v)"
  Magnitude Squared2/1 -> Add/3
  Demux/3 -> Magnitude Squared2/1
  Add/1 -> Square Root/1
  Demux/1 -> Magnitude Squared/1
  Magnitude Squared/1 -> Add/1
  Magnitude Squared1/1 -> Add/2
  Demux/2 -> Magnitude Squared1/1
  v_vec/1 -> Demux/1  "v_vec"

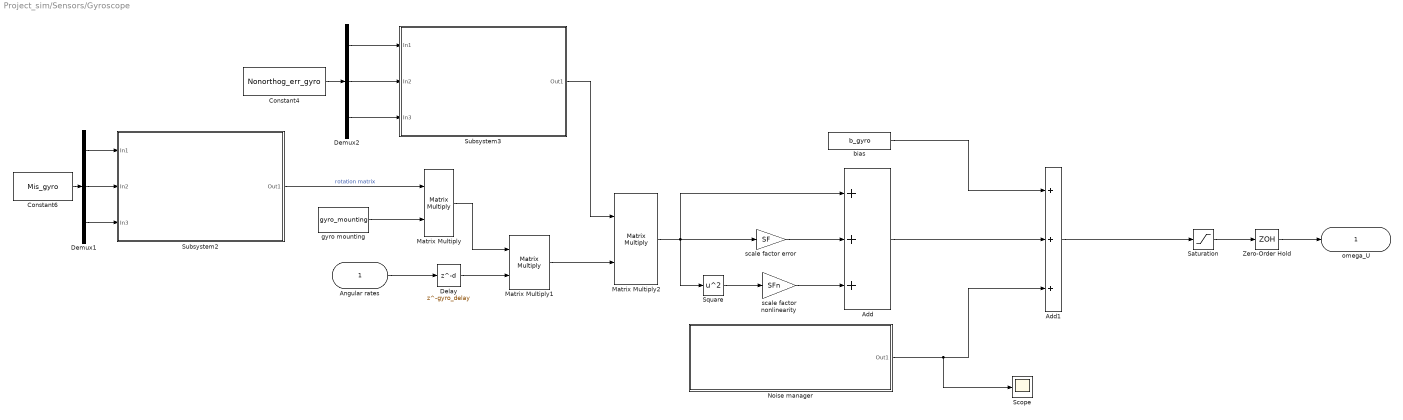
== system Project_sim/Sensors/Gyroscope ==
  Angular rates : Inport
  Add : Sum  Inputs=+++
  Add1 : Sum  Inputs=+++
  Constant4 : Constant  Value=Nonorthog_err_gyro
  Constant6 : Constant  Value=Mis_gyro
  Delay : Delay  DelayLength=gyro_delay
  Demux1 : Demux  Outputs=3
  Demux2 : Demux  Outputs=3
  Matrix Multiply : Product  Multiplication=Matrix(*)
  Matrix Multiply1 : Product  Multiplication=Matrix(*)
  Matrix Multiply2 : Product  Multiplication=Matrix(*)
  Noise manager : Subsystem
  Saturation : Saturate  UpperLimit=saturation_gyro  LowerLimit=-saturation_gyro
  Scope : Scope
      settings: ActiveDisplayYMinimum=-1  ActiveDisplayYMaximum=1  DataLoggingVariableName=ScopeData5
  Square : Math  Operator=square
  Subsystem2 : Subsystem
  Subsystem3 : Subsystem
  Zero-Order Hold : ZeroOrderHold  SampleTime=Ts_gyro
  bias : Constant  Value=b_gyro
  gyro mounting : Constant  Value=gyro_mounting
  scale factor error : Gain  Gain=SF
  scale factor nonlinearity : Gain  Gain=SFn
  omega_U : Outport
  wires:
  gyro mounting/1 -> Matrix Multiply/2
  Matrix Multiply/1 -> Matrix Multiply1/1
  Angular rates/1 -> Delay/1
  Matrix Multiply1/1 -> Matrix Multiply2/2
  Delay/1 -> Matrix Multiply1/2
  Matrix Multiply2/1 -> scale factor error/1, Add/1, Square/1
  Square/1 -> scale factor nonlinearity/1
  scale factor error/1 -> Add/2
  scale factor nonlinearity/1 -> Add/3
  Add/1 -> Add1/2
  bias/1 -> Add1/1
  Noise manager/1(Out1) -> Scope/1, Add1/3
  Add1/1 -> Saturation/1
  Saturation/1 -> Zero-Order Hold/1
  Zero-Order Hold/1 -> omega_U/1
  Demux1/1 -> Subsystem2/1(In1)
  Demux1/3 -> Subsystem2/3(In3)
  Constant4/1 -> Demux2/1
  Demux2/1 -> Subsystem3/1(In1)
  Constant6/1 -> Demux1/1
  Demux2/3 -> Subsystem3/3(In3)
  Demux1/2 -> Subsystem2/2(In2)
  Subsystem3/1(Out1) -> Matrix Multiply2/1
  Subsystem2/1(Out1) -> Matrix Multiply/1  "rotation matrix"
  Demux2/2 -> Subsystem3/2(In2)
